simulink model "TrayectoriaEvitarObstaculosPurePursuit"  (R2023b)
settings: Solver=FixedStepAuto  StartTime=0.0  StopTime=20  RelTol=1e-3  EnableMultiTasking=on
model workspace (MAT data in the model file):
  d = 0.175
libraries: robotalgslib x1
settings Model: ExtModeTrigDuration=2  Creator=Enrique  LastModifiedBy=Enrique
settings OptimizationCC: EnhancedBackFolding=on  PassReuseOutputArgsAs=Individual arguments  ZeroExternalMemoryAtStartup=off  ZeroInternalMemoryAtStartup=off  MaxStackSize=64  OptimizeBlockOrder=speed  DifferentSizesBufferReuse=on  EfficientTunableParamExpr=on
settings DebuggingCC: AlgebraicLoopMsg=none  ParameterTunabilityLossMsg=error
settings HardwareCC: ProdBitPerInt=16  ProdBitPerPointer=16  ProdBitPerSizeT=16  ProdBitPerPtrDiffT=16  ProdLargestAtomicFloat=None  ProdWordSize=8  ProdHWDeviceType=Atmel->AVR  UseEmbeddedCoderFeatures=off  UseSimulinkCoderFeatures=off
settings SFSimCC: MATLABDynamicMemAlloc=off
settings RTWCC: Description=Embedded Coder  SystemTargetFile=ert.tlc  HardwareBoard=Arduino Mega 2560  TemplateMakefile=ert_default_tmf  Toolchain=Arduino AVR  BuildConfiguration=Faster Runs
settings CodeAppCC: ForceParamTrailComments=on  IgnoreCustomStorageClasses=off  OperatorAnnotations=on  SimulinkDataObjDesc=on  SFDataObjDesc=on  InsertBlockDesc=on
settings ERTTargetCC: SupportContinuousTime=on  SupportNonInlinedSFcns=on  SupportVariableSizeSignals=on  ExtModeTransport=3  ExtModeStaticAlloc=on  ExtModeAutomaticAllocSize=off  ExtModeStaticAllocSize=2048  ExtModeMexFile=ext_xcp  ExtModeIntrfLevel=Level2 - Open

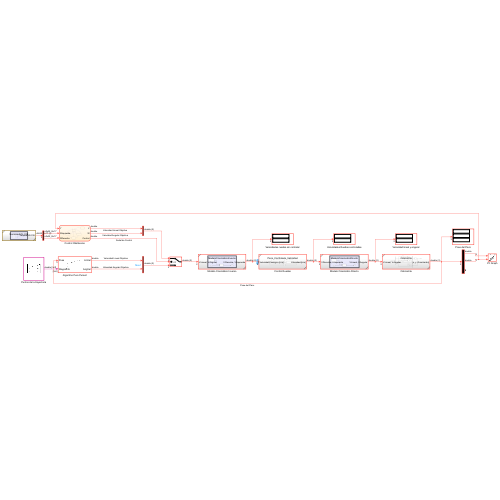
[thumbnail: Simulink's stored preview of the top-level diagram]
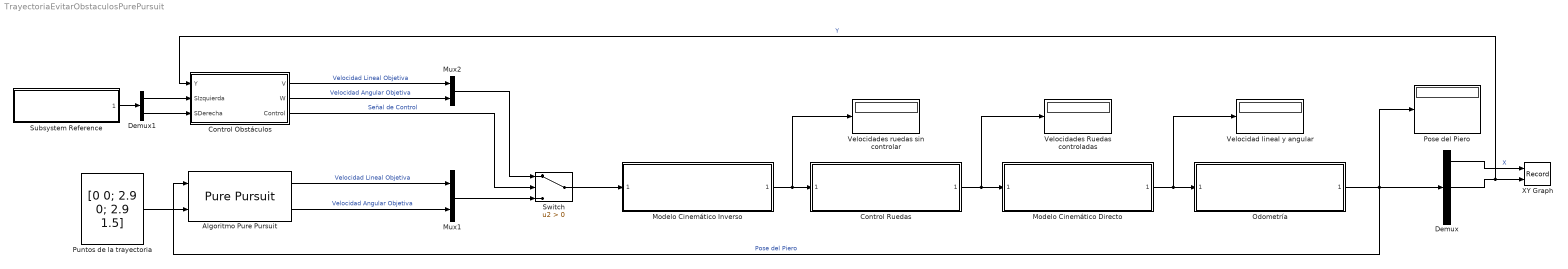
== system TrayectoriaEvitarObstaculosPurePursuit ==
  Algoritmo Pure Pursuit : robotalgslib/Pure Pursuit  DesiredLinearVelocity=0.22  MaxAngularVelocity=0.75  LookaheadDistance=0.35  TargetDirPort=off  SimulateUsing=Code generation
      settings: LibrarySourceBlock=robotmobilelib/Pure Pursuit
  Control Obstáculos : Stateflow chart  TreatAsAtomicUnit=on
  Control Ruedas : Subsystem  ReferencedSubsystem=Piero_Controlado_Velocidad
  Demux : Demux  Outputs=3
  Demux1 : Demux  Outputs=2
  Modelo Cinemático Directo : Subsystem  ReferencedSubsystem=ModeloCinematicoDirecto
  Modelo Cinemático Inverso : Subsystem  ReferencedSubsystem=ModeloCinematicoInverso
  Mux1 : Mux  Inputs=2
  Mux2 : Mux  Inputs=2
  Odometría : Subsystem  ReferencedSubsystem=Odometria
  Pose del Piero : Display
  Puntos de la trayectoria : Constant  Value=[0 0; 2.9 0; 2.9 1.5]
  Subsystem Reference : Subsystem  ReferencedSubsystem=SensoresUS_016
  Switch : Switch  Criteria=u2 > Threshold  SaturateOnIntegerOverflow=off  InputSameDT=off
  Velocidad lineal y angular : Display
  Velocidades Ruedas controladas : Display
  Velocidades ruedas sin controlar : Display
  XY Graph : Record  FileSettingsInternal="{\"entries\":[{\"content\":{\"excelSettings\":{\"content\":{},\"type\":\"Streamout.ExcelSettings\"}},\"type\":\"Streamout.FileSettingStorage\",\"uuid\":\"\"}],\"packageUris\":[\"http:\\/\\/schema.mathworks.com\\/mf0\\/streamout_blocks\\/R2020a\"],\"version\":\"1.0\"}"  Layout=[1 1]  SignalsInternal="{\"entries\":[{\"content\":{\"signals\":[{\"content\":{\"blockPath\":[],\"dimensions\":[3],\"domain\":\"\",\"hasChildren\":true,\"lineColor\":\"#77ac30\",\"port\":1,\"sid\":[\"TrayectoriaPurePursuitS:13\"],\"signalID\":1,\"signalName\":\"Pose del Piero\"},\"type\":\"RecordBlkView.Signal\",\"uuid\":\"\"},{\"content\":{\"blockPath\":[],\"channel\":[1],\"dimensions\":[3],\"domain\":\"\",\"lineColor\":\"#ff13a6\",\"parentID\":1,\"port\":1,\"sid\":[\"TrayectoriaPurePursuitS:13\"],\"signalID\":2,\"signalName\":\"Pose del Piero\"},\"type\":\"RecordBlkView.Signal\",\"uuid\":\"\"},{\"content\":{\"blockPath\":[],\"dimensions\":[1],\"domain\":\"\",\"lineColor\":\"#a2142f\",\"plots\":[ 1 ],\"port\":1,\"sid\":[\"26\"],\"signalID\":3,\"signalName\":\"X\"},\"type\":\"RecordBlkView.Signal\",\"uuid\":\"\"},{\"content\":{\"blockPath\":[],\"dimensions\":[1],\"domain\":\"\",\"lineColor\":\"#139fff\",\"plots\":[ 1 ],\"port\":2,\"sid\":[\"26\"],\"signalID\":4,\"signalName\":\"Y\"},\"type\":\"RecordBlkView.Signal\",\"uuid\":\"\"},{\"content\":{\"blockPath\":[],\"dimensions\":[2],\"domain\":\"\",\"hasChildren\":true,\"lineColor\":\"#ff6929\",\"port\":1,\"sid\":[\"TrayectoriaPurePursuitS:10\"],\"signalID\":5},\"type\":\"RecordBlkView.Signal\",\"uuid\":\"\"},{\"content\":{\"blockPath\":[],\"channel\":[1],\"dimensions\":[2],\"domain\":\"\",\"lineColor\":\"#d95319\",\"parentID\":5,\"port\":1,\"sid\":[\"TrayectoriaPurePursuitS:10\"],\"signalID\":6},\"type\":\"RecordBlkView.Signal\",\"uuid\":\"\"},{\"content\":{\"blockPath\":[],\"dimensions\":[2],\"domain\":\"\",\"hasChildren\":true,\"lineColor\":\"#64d413\",\"port\":1,\"sid\":[\"TrayectoriaPurePursuitS:11:7\"],\"signalID\":7},\"type\":\"RecordBlkView.Signal\",\"uuid\":\"\"},{\"content\":{\"blockPath\":[],\"channel\":[1],\"dimensions\":[2],\"domain\":\"\",\"lineColor\":\"#7e2f8e\",\"parentID\":7,\"port\":1,\"sid\":[\"TrayectoriaPurePursuitS:11:7\"],\"signalID\":8},\"type\":\"RecordBlkView.Signal\",\"uuid\":\"\"},{\"content\":{\"blockPath\":[],\"dimensions\":[2],\"domain\":\"\",\"hasChildren\":true,\"lineColor\":\"#fe330a\",\"port\":1,\"sid\":[\"TrayectoriaPurePursuitS:12\"],\"signalID\":9},\"type\":\"RecordBlkView.Signal\",\"uuid\":\"\"},{\"content\":{\"blockPath\":[],\"channel\":[1],\"dimensions\":[2],\"domain\":\"\",\"lineColor\":\"#4dbeee\",\"parentID\":9,\"port\":1,\"sid\":[\"TrayectoriaPurePursuitS:12\"],\"signalID\":10},\"type\":\"RecordBlkView.Signal\",\"uuid\":\"\"},{\"content\":{\"blockPath\":[],\"dimensions\":[2],\"domain\":\"\",\"hasChildren\":true,\"lineColor\":\"#0072bd\",\"port\":1,\"sid\":[\"TrayectoriaPurePursuitS:11\"],\"signalID\":11},\"type\":\"RecordBlkView.Signal\",\"uuid\":\"\"},{\"content\":{\"blockPath\":[],\"channel\":[1],\"dimensions\":[2],\"domain\":\"\",\"lineColor\":\"#139fff\",\"parentID\":11,\"port\":1,\"sid\":[\"TrayectoriaPurePursuitS:11\"],\"signalID\":12},\"type\":\"RecordBlkView.Signal\",\"uuid\":\"\"},{\"content\":{\"blockPath\":[],\"dimensions\":[2],\"domain\":\"\",\"hasChildren\":true,\"lineColor\":\"#edb120\",\"port\":1,\"sid\":[\"TrayectoriaPurePursuitS:11:6:10:4:1\"],\"signalID\":13},\"type\":\"RecordBlkView.Signal\",\"uuid\":\"\"},{\"content\":{\"blockPath\":[],\"channel\":[1],\"dimensions\":[2],\"domain\":\"\",\"lineColor\":\"#b746ff\",\"parentID\":13,\"port\":1,\"sid\":[\"TrayectoriaPurePursuitS:11:6:10:4:1\"],\"signalID\":14},\"type\":\"RecordBlkView.Signal\",\"uuid\":\"\"},{\"content\":{\"blockPath\":[],\"dimensions\":[2],\"domain\":\"\",\"hasChildren\":true,\"lineColor\":\"#77ac30\",\"port\":1,\"sid\":[\"TrayectoriaPurePursuitS:11:5\"],\"signalID\":15},\"type\":\"RecordBlkView.Signal\",\"uuid\":\"\"},{\"content\":{\"blockPath\":[],\"channel\":[1],\"dimensions\":[2],\"domain\":\"\",\"lineColor\":\"#ff13a6\",\"parentID\":15,\"port\":1,\"sid\":[\"TrayectoriaPurePursuitS:11:5\"],\"signalID\":16},\"type\":\"RecordBlkView.Signal\",\"uuid\":\"\"},{\"content\":{\"blockPath\":[],\"dimensions\":[1,1],\"domain\":\"\",\"lineColor\":\"#fe330a\",\"port\":1,\"sid\":[\"TrayectoriaPurePursuitS:11:6:10:3:34\"],\"signalID\":17},\"type\":\"RecordBlkView.Signal\",\"uuid\":\"\"},{\"content\":{\"blockPath\":[],\"dimensions\":[1,1],\"domain\":\"\",\"lineColor\":\"#22b573\",\"port\":1,\"sid\":[\"TrayectoriaPurePursuitS:11:6:10:3:38\"],\"signalID\":18},\"type\":\"RecordBlkView.Signal\",\"uuid\":\"\"},{\"content\":{\"blockPath\":[],\"dimensions\":[1,1],\"domain\":\"\",\"lineColor\":\"#0072bd\",\"port\":1,\"sid\":[\"TrayectoriaPurePursuitS:11:6:10:3:35\"],\"signalID\":19},\"type\":\"RecordBlkView.Signal\",\"uuid\":\"\"},{\"content\":{\"blockPath\":[],\"dimensions\":[1,1],\"domain\":\"\",\"lineColor\":\"#d95319\",\"port\":1,\"sid\":[\"TrayectoriaPurePursuitS:11:6:10:3:9\"],\"signalID\":20},\"type\":\"RecordBlkView.Signal\",\"uuid\":\"\"},{\"content\":{\"blockPath\":[],\"dimensions\":[1,1],\"domain\":\"\",\"lineColor\":\"#edb120\",\"port\":1,\"sid\":[\"TrayectoriaPurePursuitS:11:6:10:3:6\"],\"signalID\":21},\"type\":\"RecordBlkView.Signal\",\"uuid\":\"\"},{\"content\":{\"blockPath\":[],\"dimensions\":[1,1],\"domain\":\"\",\"lineColor\":\"#7e2f8e\",\"port\":1,\"sid\":[\"TrayectoriaPurePursuitS:11:6:10:3:1\"],\"signalID\":22},\"type\":\"RecordBlkView.Signal\",\"uuid\":\"\"},{\"content\":{\"blockPath\":[],\"dimensions\":[2],\"domain\":\"\",\"hasChildren\":true,\"lineColor\":\"#fe330a\",\"port\":1,\"sid\":[\"TrayectoriaPurePursuitS:49:6\"],\"signalID\":23},\"type\":\"RecordBlkView.Signal\",\"uuid\":\"\"},{\"content\":{\"blockPath\":[],\"channel\":[1],\"dimensions\":[2],\"domain\":\"\",\"lineColor\":\"#4dbeee\",\"parentID\":23,\"port\":1,\"sid\":[\"TrayectoriaPurePursuitS:49:6\"],\"signalID\":24},\"type\":\"RecordBlkView.Signal\",\"uuid\":\"\"},{\"content\":{\"blockPath\":[],\"dimensions\":[2],\"domain\":\"\",\"hasChildren\":true,\"lineColor\":\"#0072bd\",\"port\":1,\"sid\":[\"TrayectoriaPurePursuitS:49:4\"],\"signalID\":25},\"type\":\"RecordBlkView.Signal\",\"uuid\":\"\"},{\"content\":{\"blockPath\":[],\"channel\":[1],\"dimensions\":[2],\"domain\":\"\",\"lineColor\":\"#139fff\",\"parentID\":25,\"port\":1,\"sid\":[\"TrayectoriaPurePursuitS:49:4\"],\"signalID\":26},\"type\":\"RecordBlkView.Signal\",\"uuid\":\"\"},{\"content\":{\"blockPath\":[],\"channel\":[2],\"dimensions\":[3],\"domain\":\"\",\"lineColor\":\"#ff6929\",\"parentID\":1,\"port\":1,\"sid\":[\"TrayectoriaPurePursuitS:13\"],\"signalID\":27,\"signalName\":\"Pose del Piero\"},\"type\":\"RecordBlkView.Signal\",\"uuid\":\"\"},{\"content\":{\"blockPath\":[],\"channel\":[3],\"dimensions\":[3],\"domain\":\"\",\"lineColor\":\"#b746ff\",\"parentID\":1,\"port\":1,\"sid\":[\"TrayectoriaPurePursuitS:13\"],\"signalID\":28,\"signalName\":\"Pose del Piero\"},\"type\":\"RecordBlkView.Signal\",\"uuid\":\"\"},{\"content\":{\"blockPath\":[],\"channel\":[2],\"dimensions\":[2],\"domain\":\"\",\"lineColor\":\"#64d413\",\"parentID\":5,\"port\":1,\"sid\":[\"TrayectoriaPurePursuitS:10\"],\"signalID\":29},\"type\":\"RecordBlkView.Signal\",\"uuid\":\"\"},{\"content\":{\"blockPath\":[],\"channel\":[2],\"dimensions\":[2],\"domain\":\"\",\"lineColor\":\"#ff13a6\",\"parentID\":7,\"port\":1,\"sid\":[\"TrayectoriaPurePursuitS:11:7\"],\"signalID\":30},\"type\":\"RecordBlkView.Signal\",\"uuid\":\"\"},{\"content\":{\"blockPath\":[],\"channel\":[2],\"dimensions\":[2],\"domain\":\"\",\"lineColor\":\"#fe330a\",\"parentID\":9,\"port\":1,\"sid\":[\"TrayectoriaPurePursuitS:12\"],\"signalID\":31},\"type\":\"RecordBlkView.Signal\",\"uuid\":\"\"},{\"content\":{\"blockPath\":[],\"channel\":[2],\"dimensions\":[2],\"domain\":\"\",\"lineColor\":\"#22b573\",\"parentID\":11,\"port\":1,\"sid\":[\"TrayectoriaPurePursuitS:11\"],\"signalID\":32},\"type\":\"RecordBlkView.Signal\",\"uuid\":\"\"},{\"content\":{\"blockPath\":[],\"channel\":[2],\"dimensions\":[2],\"domain\":\"\",\"lineColor\":\"#0072bd\",\"parentID\":13,\"port\":1,\"sid\":[\"TrayectoriaPurePursuitS:11:6:10:4:1\"],\"signalID\":33},\"type\":\"RecordBlkView.Signal\",\"uuid\":\"\"},{\"content\":{\"blockPath\":[],\"channel\":[2],\"dimensions\":[2],\"domain\":\"\",\"lineColor\":\"#d95319\",\"parentID\":15,\"port\":1,\"sid\":[\"TrayectoriaPurePursuitS:11:5\"],\"signalID\":34},\"type\":\"RecordBlkView.Signal\",\"uuid\":\"\"},{\"content\":{\"blockPath\":[],\"channel\":[2],\"dimensions\":[2],\"domain\":\"\",\"lineColor\":\"#edb120\",\"parentID\":23,\"port\":1,\"sid\":[\"TrayectoriaPurePursuitS:49:6\"],\"signalID\":35},\"type\":\"RecordBlkView.Signal\",\"uuid\":\"\"},{\"content\":{\"blockPath\":[],\"channel\":[2],\"dimensions\":[2],\"domain\":\"\",\"lineColor\":\"#7e2f8e\",\"parentID\":25,\"port\":1,\"sid\":[\"TrayectoriaPurePursuitS:49:4\"],\"signalID\":36},\"type\":\"RecordBlkView.Signal\",\"uuid\":\"\"}]},\"type\":\"RecordBlkView.InputSignals\",\"uuid\":\"\"}],\"packageUris\":[\"http:\\/\\/schema.mathworks.com\\/mf0\\/streamout_blocks\\/R2020a\"],\"version\":\"1.0\"}"  VisualizationBindings="{\"xyplotplugin\":{\"info\":[{\"series\":[{\"bindingParametersList\":[{\"parameter\":\"X-Axis\",\"signalID\":3,\"signalName\":\"X\"},{\"parameter\":\"Y-Axis\",\"signalID\":4,\"signalName\":\"Y\"}],\"seriesID\":0}],\"subplotID\":1}]}}"  CompatibilityTag=XY
  wires:
  Modelo Cinemático Inverso/1 -> Velocidades ruedas sin controlar/1, Control Ruedas/1
  Control Ruedas/1 -> Velocidades Ruedas controladas/1, Modelo Cinemático Directo/1
  Modelo Cinemático Directo/1 -> Velocidad lineal y angular/1, Odometría/1
  Odometría/1 -> Pose del Piero/1, Algoritmo Pure Pursuit/1, Demux/1  "Pose del Piero"
  Demux/1 -> XY Graph/1  "X"
  Algoritmo Pure Pursuit/1 -> Mux1/1  "Velocidad Lineal Objetiva"
  Demux/2 -> Control Obstáculos/1(Y), XY Graph/2  "Y"
  Puntos de la trayectoria/1 -> Algoritmo Pure Pursuit/2
  Algoritmo Pure Pursuit/2 -> Mux1/2  "Velocidad Angular Objetiva"
  Control Obstáculos/1(V) -> Mux2/1  "Velocidad Lineal Objetiva"
  Control Obstáculos/2(W) -> Mux2/2  "Velocidad Angular Objetiva"
  Switch/1 -> Modelo Cinemático Inverso/1
  Mux1/1 -> Switch/3
  Control Obstáculos/3(Control) -> Switch/2  "Señal de Control"
  Mux2/1 -> Switch/1
  Subsystem Reference/1 -> Demux1/1
  Demux1/1 -> Control Obstáculos/2(SIzquierda)
  Demux1/2 -> Control Obstáculos/3(SDerecha)

== stateflow chart TrayectoriaEvitarObstaculosPurePursuit/Control Obstáculos ==
  state FinTrayectoria
    V=0;
    W = 0;
    Control = 1;
  state SinObstaculos
    V = 0;
    W = 0;
    Control = 0;
  state ObstaculoIzquierda
    V = 0.1;
    W = -pi/4;
    Control = 1;
  state ObstaculoDerecha
    V = 0.1;
    W = pi/4;
    Control = 1;
  state ObstaculoFrente
    V = 0;
    W = pi/2;
    Control = 1;
  SinObstaculos -> FinTrayectoria [order 3] : [Y > 1]
  (default) -> SinObstaculos
  SinObstaculos -> ObstaculoIzquierda [order 1] : [SIzquierda < 30]
  SinObstaculos -> ObstaculoDerecha [order 2] : [SDerecha < 30]
  ObstaculoIzquierda -> SinObstaculos [order 1] : [after(1,sec)]
  ObstaculoFrente -> SinObstaculos : [after(1.5,sec)]
  ObstaculoDerecha -> SinObstaculos [order 1] : [after(1,sec)]
  ObstaculoIzquierda -> ObstaculoFrente [order 2] : [SDerecha < 15]
  ObstaculoDerecha -> ObstaculoFrente [order 2] : [SIzquierda < 15]
  data: Y input; V output; W output; Control output; SIzquierda input; SDerecha input
